simulink model "heli_master"  (R2018b)
settings: Solver=ode1  StartTime=0.0  StopTime=10  FixedStep=0.002  RelTol=1e-3  EnableMultiTasking=on
PostLoadFcn:
  | qc_set_target_type(getConfigSet(bdroot, 'QUARC Default Target Configuration'));
undefined symbols (not defined in the file or in its folder): HIL, qc_get_step_size
libraries: simulink_extras x5, quarc_library x3
settings Model: ExtModeTrigDuration=5000  Creator=Rchan  LastModifiedBy=Robert
settings SolverCC: PositivePriorityOrder=on
settings DataIOCC: LimitDataPoints=on  SaveFormat=Array  SignalLoggingSaveFormat=ModelDataLogs
settings OptimizationCC: ExpressionDepthLimit=2147483647  InitFltsAndDblsToZero=on  LifeSpan=inf
settings DebuggingCC: SaveWithParameterizedLinksMsg=none  UnderspecifiedInitializationDetection=Classic  MergeDetectMultiDrivingBlocksExec=none  SolverPrmCheckMsg=warning  MultiTaskDSMMsg=warning  MultiTaskCondExecSysMsg=none  FcnCallInpInsideContextMsg=warning  StateNameClashWarn=warning  SFUnexpectedBacktrackingDiag=warning  SFNoUnconditionalDefaultTransitionDiag=warning  SFExecutionAtInitializationDiag=none
settings HardwareCC: ProdBitPerPointer=32  ProdBitPerSizeT=32  ProdBitPerPtrDiffT=32  ProdLargestAtomicFloat=None  ProdIntDivRoundTo=Undefined  ProdEndianess=Unspecified  ProdWordSize=32  ProdHWDeviceType=32-bit Generic
settings ModelReferenceCC: PropagateSignalLabelsOutOfModel=off
settings SFSimCC: SimUseLocalCustomCode=off
settings RTWCC: SystemTargetFile=quarc_win64.tlc  TemplateMakefile=quarc_default_tmf  Description=QUARC Win64 Target  RTWUseLocalCustomCode=off
settings CodeAppCC: StateflowObjectComments=on
settings STFCustomTargetCC: TargetPreCompLibLocation=D:\PROGRA~3\QUARC\lib\2014a\win64\release  ConcurrentExecutionCompliant=on  GeneratePreprocessorConditionals=Disable all  CPPClassGenCompliant=on  GRTInterface=on  SystemTargetFile=quarc_win64.tlc
settings GRTTargetCC: TargetPreCompLibLocation=D:\PROGRA~3\QUARC\lib\2014a\win64\release  TargetLangStandard=C89/C90 (ANSI)  ParMdlRefBuildCompliant=off  CompOptLevelCompliant=off  GeneratePreprocessorConditionals=Disable all  CombineOutputUpdateFcns=off  MatFileLogging=off  GRTInterface=on  UseToolchainInfoCompliant=off  ExtMode=on  ExtModeMexFile=quarc_comm
settings ConfigComp: CovMetricSettings=dw  CovHtmlReporting=on  CovSaveCumulativeToWorkspaceVar=on  CovSaveSingleToWorkspaceVar=on  CovExternalEMLEnable=off  CovSFcnEnable=off

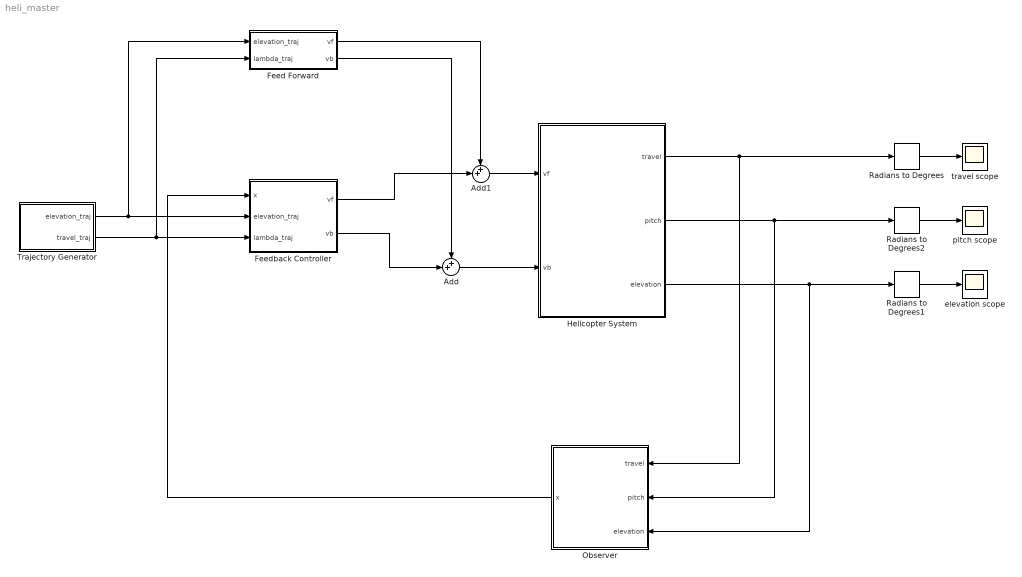
== system heli_master ==
  Add : Sum  Inputs=++|
  Add1 : Sum  Inputs=++|
  Feed Forward : Subsystem
  Feedback Controller : Subsystem
  Helicopter System : Subsystem  Variant=on
  Observer : Subsystem
  Radians to Degrees : simulink_extras/Transformations/Radians to Degrees
  Radians to Degrees1 : simulink_extras/Transformations/Radians to Degrees
  Radians to Degrees2 : simulink_extras/Transformations/Radians to Degrees
  Trajectory Generator : Subsystem
  elevation scope : Scope
  pitch scope : Scope
  travel scope : Scope
  wires:
  Helicopter System/1(travel) -> Observer/1(travel), Radians to Degrees/1
  Helicopter System/3(elevation) -> Observer/3(elevation), Radians to Degrees1/1
  Helicopter System/2(pitch) -> Observer/2(pitch), Radians to Degrees2/1
  Radians to Degrees/1 -> travel scope/1
  Radians to Degrees2/1 -> pitch scope/1
  Radians to Degrees1/1 -> elevation scope/1
  Add/1 -> Helicopter System/2(vb)
  Add1/1 -> Helicopter System/1(vf)
  Feed Forward/1(vf) -> Add1/1
  Feed Forward/2(vb) -> Add/1
  Feedback Controller/1(vf) -> Add1/2
  Feedback Controller/2(vb) -> Add/2
  Observer/1(x) -> Feedback Controller/1(x)
  Trajectory Generator/1(elevation_traj) -> Feed Forward/1(elevation_traj), Feedback Controller/2(elevation_traj)
  Trajectory Generator/2(travel_traj) -> Feed Forward/2(lambda_traj), Feedback Controller/3(lambda_traj)

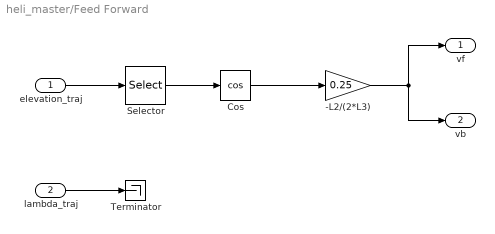
== system heli_master/Feed Forward ==
  elevation_traj : Inport
  lambda_traj : Inport  Port=2
  -L2/(2*L3) : Gain  Gain=0.25
  Cos : Trigonometry  Operator=cos
  Selector : Selector  InputPortWidth=5  IndexOptions=Index vector (dialog)  Indices=1  OutputSizes=1
  Terminator : Terminator
  vf : Outport
  vb : Outport  Port=2
  wires:
  lambda_traj/1 -> Terminator/1
  elevation_traj/1 -> Selector/1
  Selector/1 -> Cos/1
  Cos/1 -> -L2/(2*L3)/1
  -L2/(2*L3)/1 -> vb/1, vf/1

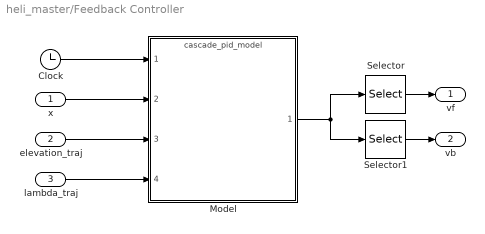
== system heli_master/Feedback Controller ==
  x : Inport
  elevation_traj : Inport  Port=2
  lambda_traj : Inport  Port=3
  Clock : Clock
  Model : ModelReference  ModelNameDialog=cascade_pid_model  SimulationMode=Normal  ModelReferenceVersion=1.6
  Selector : Selector  InputPortWidth=2  IndexOptions=Index vector (dialog)  Indices=1  OutputSizes=1
  Selector1 : Selector  InputPortWidth=2  IndexOptions=Index vector (dialog)  Indices=2  OutputSizes=1
  vf : Outport
  vb : Outport  Port=2
  wires:
  Clock/1 -> Model/1
  x/1 -> Model/2
  elevation_traj/1 -> Model/3
  lambda_traj/1 -> Model/4
  Selector/1 -> vf/1
  Selector1/1 -> vb/1
  Model/1 -> Selector1/1, Selector/1

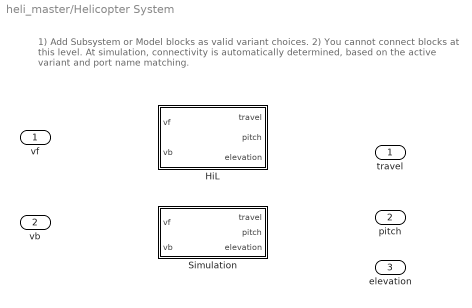
== system heli_master/Helicopter System ==
  note: 1) Add Subsystem or Model blocks as valid variant choices.
      | 2) You cannot connect blocks at this level. At simulation, connectivity is automatically
      | determined, based on the active variant and port name matching.
  vf : Inport
  vb : Inport  Port=2
  HiL : Subsystem  VariantControl=variant_hil == true
  Simulation : Subsystem  VariantControl=variant_hil == false
  travel : Outport
  pitch : Outport  Port=2
  elevation : Outport  Port=3

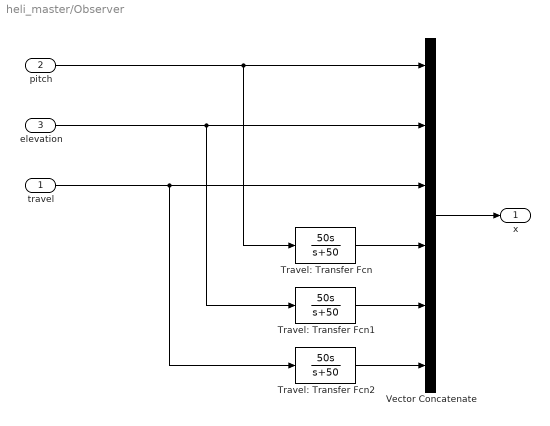
== system heli_master/Observer ==
  travel : Inport
  pitch : Inport  Port=2
  elevation : Inport  Port=3
  Travel: Transfer Fcn : TransferFcn  Numerator=[50 0]  Denominator=[1 50]
  Travel: Transfer Fcn1 : TransferFcn  Numerator=[50 0]  Denominator=[1 50]
  Travel: Transfer Fcn2 : TransferFcn  Numerator=[50 0]  Denominator=[1 50]
  Vector Concatenate : Concatenate  NumInputs=6
  x : Outport
  wires:
  pitch/1 -> Vector Concatenate/1, Travel: Transfer Fcn/1
  elevation/1 -> Vector Concatenate/2, Travel: Transfer Fcn1/1
  travel/1 -> Vector Concatenate/3, Travel: Transfer Fcn2/1
  Vector Concatenate/1 -> x/1
  Travel: Transfer Fcn/1 -> Vector Concatenate/4
  Travel: Transfer Fcn1/1 -> Vector Concatenate/5
  Travel: Transfer Fcn2/1 -> Vector Concatenate/6

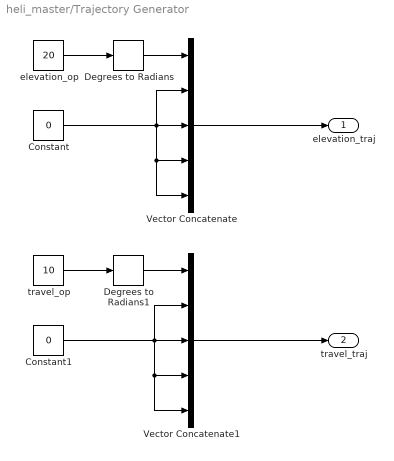
== system heli_master/Trajectory Generator ==
  Constant : Constant  Value=0
  Constant1 : Constant  Value=0
  Degrees to Radians : simulink_extras/Transformations/Degrees to Radians
  Degrees to Radians1 : simulink_extras/Transformations/Degrees to Radians
  Vector Concatenate : Concatenate  NumInputs=5
  Vector Concatenate1 : Concatenate  NumInputs=5
  elevation_op : Constant  Value=20
  travel_op : Constant  Value=10
  elevation_traj : Outport
  travel_traj : Outport  Port=2
  wires:
  Vector Concatenate/1 -> elevation_traj/1
  Vector Concatenate1/1 -> travel_traj/1
  Constant/1 -> Vector Concatenate/2, Vector Concatenate/3, Vector Concatenate/5, Vector Concatenate/4
  Constant1/1 -> Vector Concatenate1/3, Vector Concatenate1/2, Vector Concatenate1/4, Vector Concatenate1/5
  elevation_op/1 -> Degrees to Radians/1
  Degrees to Radians/1 -> Vector Concatenate/1
  travel_op/1 -> Degrees to Radians1/1
  Degrees to Radians1/1 -> Vector Concatenate1/1

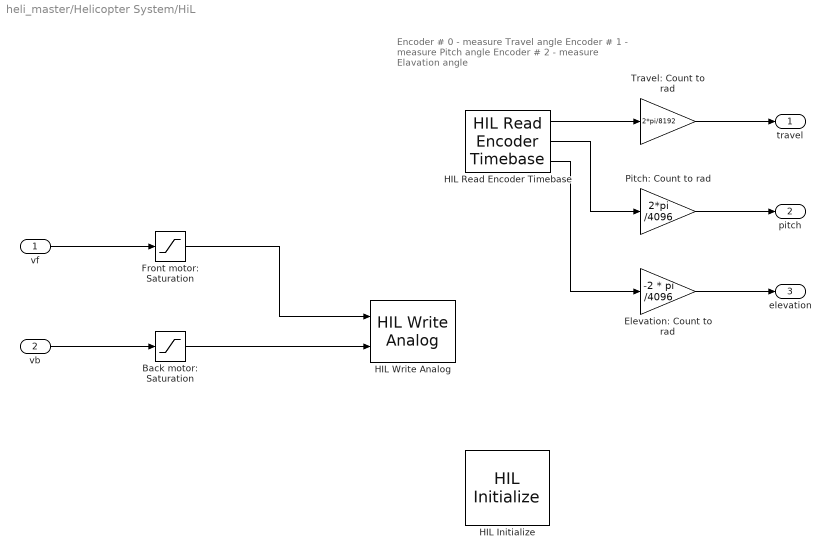
== system heli_master/Helicopter System/HiL ==
  note: Encoder # 0 - measure Travel angle
      | Encoder # 1 - measure Pitch angle
      | Encoder # 2 - measure Elavation angle
  vf : Inport
  vb : Inport  Port=2
  Back motor: Saturation : Saturate  UpperLimit=5  LowerLimit=-5
  Elevation: Count to rad : Gain  Gain=-2 * pi /4096
  Front motor: Saturation : Saturate  UpperLimit=5  LowerLimit=-5
  HIL Initialize : quarc_library/Data Acquisition/Generic/Configuration/HIL Initialize  Priority=-99  object_name=HIL-1  board_type=q8_usb  board_number=0  board_options=update_rate=normal;decimation=1  exclusive=off  active=off  hardware_clocks=[0:2]  clock_modes=[]  initial_clock_frequencies=[]  set_clock_params_at_start=off  set_clock_params_at_switch_in=off  set_clock_frequencies_at_start=off  set_clock_frequencies_at_switch_in=off  analog_input_channels=[0:7]  analog_input_maximums=10  analog_input_minimums=-10  set_analog_input_params_at_start=on  set_analog_input_params_at_switch_in=off  analog_output_channels=[0:7]  analog_output_maximums=10  analog_output_minimums=-10  initial_analog_outputs=[0]  final_analog_outputs=[0]  watchdog_analog_outputs=0  set_analog_output_params_at_start=on  set_analog_output_params_at_switch_in=off  set_analog_outputs_at_start=on  set_analog_outputs_at_switch_in=off  set_analog_outputs_at_terminate=on  set_analog_outputs_at_switch_out=off  set_analog_outputs_on_watchdog=off  digital_input_channels=[]  digital_output_channels=[]  digital_output_configuration=[]  initial_digital_outputs=[1]  final_digital_outputs=[1]  watchdog_digital_outputs=[1]  set_digital_output_params_at_start=off  set_digital_output_params_at_switch_in=off  set_digital_outputs_at_start=on  set_digital_outputs_at_switch_in=off  set_digital_outputs_at_terminate=on  set_digital_outputs_at_switch_out=off  set_digital_outputs_on_watchdog=off  encoder_channels=[0:7]  quadrature=[4]  encoder_filter_frequency=[]  initial_encoder_counts=[0]  set_encoder_params_at_start=on  set_encoder_params_at_switch_in=off  set_encoder_counts_at_start=on  set_encoder_counts_at_switch_in=off  pwm_channels=[0:7]  pwm_modes=0  pwm_frequency=99.532799999999995e6/4095  pwm_configuration=[0]  pwm_alignment=[0]  pwm_polarity=[1]  pwm_leading_deadband=[0]  pwm_trailing_deadband=[0]  initial_pwm_outputs=[0]  final_pwm_outputs=[0]  watchdog_pwm_outputs=[0]  set_pwm_params_at_start=on  set_pwm_params_at_switch_in=off  set_pwm_outputs_at_start=on  set_pwm_outputs_at_switch_in=off  set_pwm_outputs_at_terminate=on  set_pwm_outputs_at_switch_out=off  set_pwm_outputs_on_watchdog=off  other_output_channels=[]  initial_other_outputs=[]  final_other_outputs=[]  watchdog_other_outputs=[]  set_other_outputs_at_start=off  set_other_outputs_at_switch_in=off  set_other_outputs_at_terminate=off  set_other_outputs_at_switch_out=off  set_other_outputs_on_watchdog=off
  HIL Read Encoder Timebase : quarc_library/Data Acquisition/Generic/Timebases/HIL Read Encoder Timebase  object_name=HIL-1  clock=0  channels=[0:2]  samples_in_buffer=max(ceil(1/qc_get_step_size), 1)  active=on  vector_output=off  data_type_mode=Inherit via back propagation  data_type=double
  HIL Write Analog : quarc_library/Data Acquisition/Generic/Immediate I//O/HIL Write Analog  object_name=HIL-1  channels=[0:1]  sample_time=-1  active=off  vector_input=off
  Pitch: Count to rad : Gain  Gain=2*pi /4096
  Travel: Count to rad : Gain  Gain=2*pi/8192
  travel : Outport
  pitch : Outport  Port=2
  elevation : Outport  Port=3
  wires:
  vf/1 -> Front motor: Saturation/1
  vb/1 -> Back motor: Saturation/1
  Back motor: Saturation/1 -> HIL Write Analog/2
  HIL Read Encoder Timebase/2 -> Pitch: Count to rad/1
  HIL Read Encoder Timebase/1 -> Travel: Count to rad/1
  Front motor: Saturation/1 -> HIL Write Analog/1
  HIL Read Encoder Timebase/3 -> Elevation: Count to rad/1
  Travel: Count to rad/1 -> travel/1
  Pitch: Count to rad/1 -> pitch/1
  Elevation: Count to rad/1 -> elevation/1

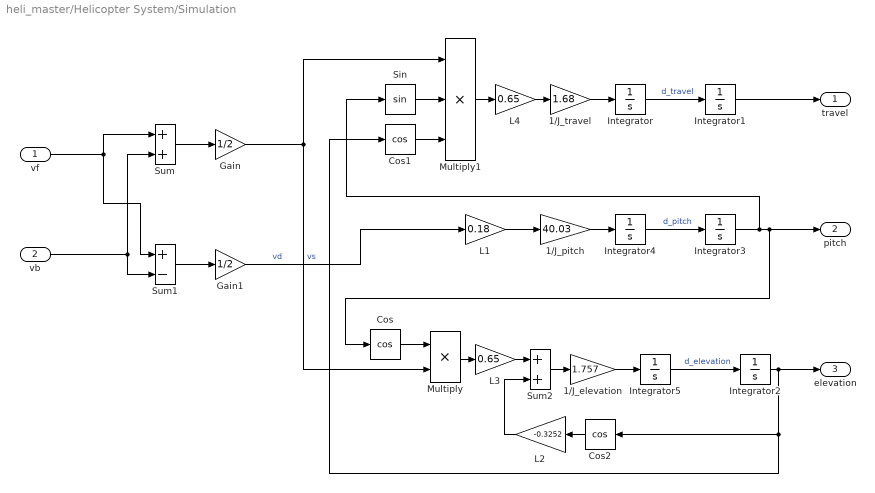
== system heli_master/Helicopter System/Simulation ==
  vf : Inport
  vb : Inport  Port=2
  1/J_elevation : Gain  Gain=1.757
  1/J_pitch : Gain  Gain=40.03
  1/J_travel : Gain  Gain=1.68
  Cos : Trigonometry  Operator=cos
  Cos1 : Trigonometry  Operator=cos
  Cos2 : Trigonometry  Operator=cos
  Gain : Gain  Gain=1/2
  Gain1 : Gain  Gain=1/2
  Integrator : Integrator
  Integrator1 : Integrator  LimitOutput=on  UpperSaturationLimit=2.1  LowerSaturationLimit=-2.1
  Integrator2 : Integrator  LimitOutput=on  UpperSaturationLimit=1.22  LowerSaturationLimit=-1.22
  Integrator3 : Integrator  LimitOutput=on  UpperSaturationLimit=1.4  LowerSaturationLimit=-1.4
  Integrator4 : Integrator
  Integrator5 : Integrator
  L1 : Gain  Gain=0.18
  L2 : Gain  Gain=-0.3252
  L3 : Gain  Gain=0.65
  L4 : Gain  Gain=0.65
  Multiply : Product
  Multiply1 : Product  Inputs=3
  Sin : Trigonometry
  Sum : Sum
  Sum1 : Sum  Inputs=+-
  Sum2 : Sum
  travel : Outport
  pitch : Outport  Port=2
  elevation : Outport  Port=3
  wires:
  Integrator/1 -> Integrator1/1  "d_travel"
  Integrator1/1 -> travel/1
  Integrator3/1 -> Sin/1, Cos/1, pitch/1
  Integrator4/1 -> Integrator3/1  "d_pitch"
  Integrator2/1 -> Cos2/1, Cos1/1, elevation/1
  Integrator5/1 -> Integrator2/1  "d_elevation"
  vf/1 -> Sum/1, Sum1/1
  vb/1 -> Sum1/2, Sum/2
  Sum/1 -> Gain/1
  Sum1/1 -> Gain1/1
  1/J_pitch/1 -> Integrator4/1
  L1/1 -> 1/J_pitch/1
  Gain1/1 -> L1/1  "vd"
  Cos/1 -> Multiply/1
  Gain/1 -> Multiply1/1, Multiply/2  "vs"
  1/J_elevation/1 -> Integrator5/1
  1/J_travel/1 -> Integrator/1
  Multiply/1 -> L3/1
  Multiply1/1 -> L4/1
  L4/1 -> 1/J_travel/1
  Sin/1 -> Multiply1/2
  Cos1/1 -> Multiply1/3
  Sum2/1 -> 1/J_elevation/1
  L3/1 -> Sum2/1
  L2/1 -> Sum2/2
  Cos2/1 -> L2/1
